simulink library "Actuator_Lib2"  (R2013a)
settings: Solver=ode45  StartTime=0.0  StopTime=10.0  RelTol=1e-3
values from neighbouring files (symbols this model uses):
  AC = FASER_config    [UAV_config.m]    (also in UAV_modelconfig.mat = )
  TrimCondition =     [UAV_trimcondition.mat]
undefined symbols (not defined in the file or in its folder): SampleTime
libraries: simulink x9, Actuator_Lib x6
settings Model: Creator=austinmurch  LastModifiedBy=descobar

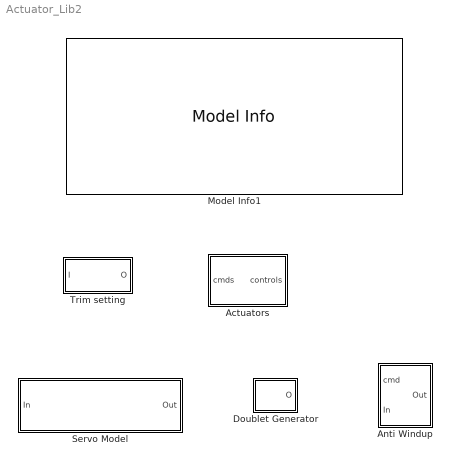
== system Actuator_Lib2 ==
  Actuators : Subsystem
  Anti Windup : Subsystem  mask(Integrator Anti-Windup){MAX_DEF=0, MIN_DEF=0, gain_sign=off}
      mask prompts: MAX_DEF "Maximum surface deflection limit"; MIN_DEF "Minimum surface deflection limit"; gain_sign "Positive gains in control law"
      mask help:
      | This block uses boolean logic to eliminate integrator windup.
      | It compares the sign of the error between reference and output,
      | and the sign and position of the surface being controlled.
      mask Help:
      | See the "READ ME" block under the mask for a more thorough explanation of
      | how this block works.
  Doublet Generator : Subsystem  mask(DoubletGenerator){timeon=[3 10 17], pulsewidth=[2 2 2], amplitude=[0 0 0]}
      mask prompts: timeon "Time Start"; pulsewidth "Pulse Duration"
      mask help:
      | Doublet Generator.
      | Ouputs doublet of specificed amplitude and duration.
      |
      | If start/duration/amplitude parameters are vectors, then output is multichannel.
      mask Display: plot([.1 .3 .3001 .4 .4001 .5  .5001 .7],[0 0 1 1 -1 -1 0 0])
  Model Info1 : simulink/Model-Wide Utilities/Model Info  InitialBlockCM=None  BlockCM=None  Frame=on  DisplayStringWithTags=|  HorizontalTextAlignment=Left  LeftAlignmentValue=0.02  SourceBlockDiagram=Actuator_Lib  TagMaxNumber=20
      | MODEL INFORMATION
      | Actuator Model Library
      | 
      | University of Minnesota
      | Aerospace Engineering and Mechanics
      | Copyright 2011 Regents of the University of Minnesota. All rights reserved.
      | 
      | == SVN Info ==
      | %<ModelVersion>
      | Last modified by %<LastModifiedBy> on %<LastModificationDate>
  Servo Model : Subsystem  mask(Rate and Position Limited Servo){freq=10, RL=999.0, POS_hi=20.0, POS_lo=-30.0}
      mask prompts: freq "Bandwidth, Hz"; RL "Rate Limit:"; POS_hi "Position Limit High:"; POS_lo "Position Limit Low:"
      mask help: First order transfer function: w/(s+w), with rate and position limits.
      mask Help:
      | This block models a first order servo with the initial condition
      | on the integrator set to the steady state value for constant input.
      | The servo is rate and position limited and those values are set
      | in the block parameters.
      mask Display:
      | text(.48,.55,sprintf('%3.1f Hz\nBW',freq),'horizontalAlignment','center');
      | 
      | text(0.18,0.45,sprintf('|d/dt|\n<%0.1f',RL),'horizontalAlignment','center');
      | 
      | text(0.88,0.85,num2str(POS_hi),'horizontalAlignment', 'center');
      | text(0.88,0.2,num2str(POS_lo),'horizontalAlignment', 'center');
      | text(0.73,0.5,'P\nL');
      | 
      | 
      | plot([0.83 0.87 0.93 0.97],[0.4 0.4 0.6 0.6]);
      | plot([0.81 0.99],[0.5 0.5]);
      | plot([0.9 0.9],[0.3 0.7]);
      | plot([0.81 0.99 0.99 0.81 0.81],[0.3 0.3 0.7 0.7 0.3]);
  "Trim setting " : Subsystem

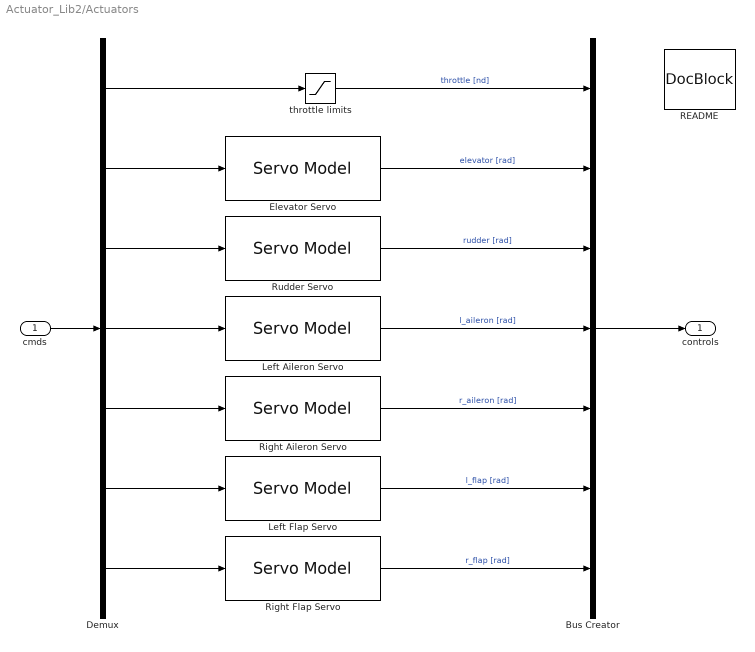
== system Actuator_Lib2/Actuators ==
  cmds : Inport
  Bus Creator : BusCreator  Inputs=7
  Demux : Demux  Outputs=7
  Elevator Servo : Actuator_Lib/Servo Model  freq=AC.Actuator.elevator.BW  RL=AC.Actuator.elevator.RateLim  POS_hi=AC.Actuator.elevator.PosLim  POS_lo=AC.Actuator.elevator.NegLim
  Left Aileron Servo : Actuator_Lib/Servo Model  freq=AC.Actuator.l_aileron.BW  RL=AC.Actuator.l_aileron.RateLim  POS_hi=AC.Actuator.l_aileron.PosLim  POS_lo=AC.Actuator.l_aileron.NegLim
  Left Flap Servo : Actuator_Lib/Servo Model  freq=AC.Actuator.l_flap.BW  RL=AC.Actuator.l_flap.RateLim  POS_hi=AC.Actuator.l_flap.PosLim  POS_lo=AC.Actuator.l_flap.NegLim
  README : simulink/Model-Wide Utilities/DocBlock  DocumentType=Text
      content=|
      | Actuators
      |
      | This block implements first order, rate and position limited actuator
      | models for the aileron, elevator, rudder and flap channels. The throttle
      | does not have a servo, but is position limited.
      |
      | Parameters for these models are contained in the aircraft configuration
      | data structure variable, "AC". Specfically,
      |
      | >> AC.Actuator
      |
      | ans =
      |
      |      elevator: [1x1 struct]
      |     l_aileron: [1x1 struct]
      |     r_aileron: [1x1 struct]
      |        rudder: [1x1 struct]
      |        l_flap: [1x1 struct]
      |        r_flap: [1x1 struct]
      |      throttle: [1x1 struct]
      |
      | Control Inputs Sign Convention
      | Elevator: +TED
      | Rudder: +TEL
      | Ailerons: +TED, da = (da_R-da_L)/2
      | Flaps: +TED
      | Throttle: always positive
  Right Aileron Servo : Actuator_Lib/Servo Model  freq=AC.Actuator.r_aileron.BW  RL=AC.Actuator.r_aileron.RateLim  POS_hi=AC.Actuator.r_aileron.PosLim  POS_lo=AC.Actuator.r_aileron.NegLim
  Right Flap Servo : Actuator_Lib/Servo Model  freq=AC.Actuator.l_flap.BW  RL=AC.Actuator.l_flap.RateLim  POS_hi=AC.Actuator.l_flap.PosLim  POS_lo=AC.Actuator.l_flap.NegLim
  Rudder Servo : Actuator_Lib/Servo Model  freq=AC.Actuator.rudder.BW  RL=AC.Actuator.rudder.RateLim  POS_hi=AC.Actuator.rudder.PosLim  POS_lo=AC.Actuator.rudder.NegLim
  throttle limits : Saturate  UpperLimit=AC.Actuator.throttle.PosLim  LowerLimit=AC.Actuator.throttle.NegLim
  controls : Outport
  wires:
  Demux/5 -> Right Aileron Servo/1
  Demux/7 -> Right Flap Servo/1
  Right Flap Servo/1 -> Bus Creator/7  "r_flap [rad]"
  Right Aileron Servo/1 -> Bus Creator/5  "r_aileron [rad]"
  Left Flap Servo/1 -> Bus Creator/6  "l_flap [rad]"
  Demux/6 -> Left Flap Servo/1
  Left Aileron Servo/1 -> Bus Creator/4  "l_aileron [rad]"
  Demux/4 -> Left Aileron Servo/1
  Rudder Servo/1 -> Bus Creator/3  "rudder [rad]"
  Demux/3 -> Rudder Servo/1
  Elevator Servo/1 -> Bus Creator/2  "elevator [rad]"
  Demux/2 -> Elevator Servo/1
  throttle limits/1 -> Bus Creator/1  "throttle [nd]"
  Demux/1 -> throttle limits/1
  cmds/1 -> Demux/1
  Bus Creator/1 -> controls/1

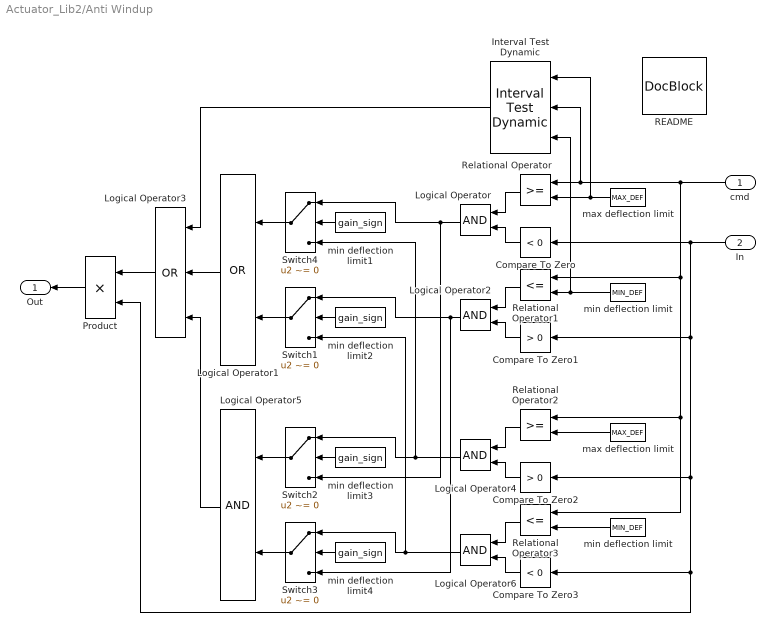
== system Actuator_Lib2/Anti Windup ==
  cmd : Inport
  In : Inport  Port=2
  Compare To Zero : simulink/Logic and Bit Operations/Compare To Zero  SystemSampleTime=-1  relop=<  LogicOutDataTypeMode=uint8
  Compare To Zero1 : simulink/Logic and Bit Operations/Compare To Zero  SystemSampleTime=-1  relop=>  LogicOutDataTypeMode=uint8
  Compare To Zero2 : simulink/Logic and Bit Operations/Compare To Zero  SystemSampleTime=-1  relop=>  LogicOutDataTypeMode=uint8
  Compare To Zero3 : simulink/Logic and Bit Operations/Compare To Zero  SystemSampleTime=-1  relop=<  LogicOutDataTypeMode=uint8
  Interval Test Dynamic : simulink/Logic and Bit Operations/Interval Test Dynamic  SystemSampleTime=-1  IntervalClosedRight=on  IntervalClosedLeft=on  LogicOutDataTypeMode=boolean
  Logical Operator{,2,4..6} (5 alike) : Logic  AllPortsSameDT=off  OutDataTypeStr=boolean  SampleTime=SampleTime
  Logical Operator1 : Logic  Operator=OR  AllPortsSameDT=off  OutDataTypeStr=boolean  SampleTime=SampleTime
  Logical Operator3 : Logic  Operator=OR  Inputs=3  AllPortsSameDT=off  OutDataTypeStr=boolean  SampleTime=SampleTime
  Product : Product  RndMeth=Zero
  README : simulink/Model-Wide Utilities/DocBlock  SystemSampleTime=-1  DocumentType=Text
      content=|
      | This block uses anti-windup logic to either stop or continue integrating.
      |
      | The first input signal, 'cmd', must come from the control surface command
      | that is the output of the controller. For instance, if the outputs of a PI
      | control phi tracker (with anti-windup) and a P control roll damper are
      | summed and sent to the aileron command, then the summed value must be fed
      | back into the 'cmd' input of this anti-windup block, as opposed to just the
      | output of the phi tracker.
      |
      | The second input signal, 'In', must come from the error that is being fed
      | into the control law.
      |
      | The output signal, 'Out' must feed into the error integrator block.
      |
      | For the anti-windup to work as intended, a saturation block must be placed
      | on the ouput of the control command being fed to the associated actuator.
      | If the controller is in delta coordinates, the limits in the saturation
      | block must be the actuator limits minus the trimmed control surface value.
      | For instance, for and aileron command, the limits would be:
      | Upper Limit: AC.Actuator.r_aileron.PosLim-TrimCondition.Inputs.r_aileron
      | Lower Limit: AC.Actuator.r_aileron.NegLim-TrimCondition.Inputs.r_aileron
      |
      | Depending on which surface is being controlled, the windup logic may
      | change. The default logic for this block is the following:
      |
      | For input u, saturation limits Umax and Umin, and error e,
      | If u is in bounds, do nothing
      | If u >= Umax AND e < 0, stop integrating
      | If u >= Umax AND e > 0, continue integrating
      | If u <= Umin AND e < 0, continue integrating
      | If u <= Umin AND e > 0, stop integrating
      |
      | This is the logic for a plant transfer function with a negative gain. In
      | other words, a positive input gives a negative response, which is usually
      | the case with flight dynamics. If the plant transfer function does not have
      | a negative gain, the logic will need to be reversed. In this case, the
      | inequalities on the error logic must be switched, so
      | If u is in bounds, do nothing
      | If u >= Umax AND e > 0, stop integrating
      | If u >= Umax AND e < 0, continue integrating
      | If u <= Umin AND e > 0, continue integrating
      | If u <= Umin AND e < 0, stop integrating
  Relational Operator : RelationalOperator  OutDataTypeStr=boolean
  Relational Operator1 : RelationalOperator  Operator=<=  OutDataTypeStr=boolean
  Relational Operator2 : RelationalOperator  OutDataTypeStr=boolean
  Relational Operator3 : RelationalOperator  Operator=<=  OutDataTypeStr=boolean
  Switch{1..4} (4 alike) : Switch  Criteria=u2 ~= 0  SampleTime=SampleTime
  max deflection limit : Constant  Value=MAX_DEF  SampleTime=SampleTime
  "max deflection limit " : Constant  Value=MAX_DEF  SampleTime=SampleTime
  min deflection limit : Constant  Value=MIN_DEF  SampleTime=SampleTime
  "min deflection limit " : Constant  Value=MIN_DEF  SampleTime=SampleTime
  min deflection limit{1..4} (4 alike) : Constant  Value=gain_sign  SampleTime=SampleTime
  Out : Outport
  wires:
  Logical Operator5/1 -> Logical Operator3/3
  "max deflection limit "/1 -> Relational Operator2/2
  "min deflection limit "/1 -> Relational Operator3/2
  Relational Operator3/1 -> Logical Operator6/1
  Compare To Zero3/1 -> Logical Operator6/2
  Relational Operator2/1 -> Logical Operator4/1
  Compare To Zero2/1 -> Logical Operator4/2
  Interval Test Dynamic/1 -> Logical Operator3/1
  Logical Operator1/1 -> Logical Operator3/2
  Logical Operator3/1 -> Product/1
  Product/1 -> Out/1
  min deflection limit/1 -> Interval Test Dynamic/3, Relational Operator1/2
  Relational Operator1/1 -> Logical Operator2/1
  Compare To Zero1/1 -> Logical Operator2/2
  In/1 -> Product/2, Compare To Zero3/1, Compare To Zero2/1, Compare To Zero1/1, Compare To Zero/1
  Relational Operator/1 -> Logical Operator/1
  Compare To Zero/1 -> Logical Operator/2
  cmd/1 -> Relational Operator3/1, Relational Operator2/1, Relational Operator1/1, Interval Test Dynamic/2, Relational Operator/1
  max deflection limit/1 -> Interval Test Dynamic/1, Relational Operator/2
  min deflection limit2/1 -> Switch1/2
  min deflection limit3/1 -> Switch2/2
  min deflection limit4/1 -> Switch3/2
  Switch2/1 -> Logical Operator5/1
  Switch3/1 -> Logical Operator5/2
  Switch1/1 -> Logical Operator1/2
  Switch4/1 -> Logical Operator1/1
  min deflection limit1/1 -> Switch4/2
  Logical Operator/1 -> Switch4/1, Switch2/3
  Logical Operator2/1 -> Switch1/1, Switch3/3
  Logical Operator4/1 -> Switch2/1, Switch4/3
  Logical Operator6/1 -> Switch3/1, Switch1/3

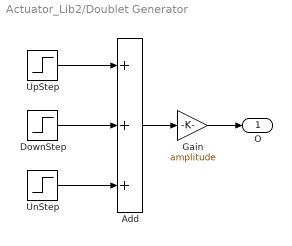
== system Actuator_Lib2/Doublet Generator ==
  Add : Sum  Inputs=+++
  DownStep : Step  Time=timeon+pulsewidth  After=-2  SampleTime=0
  Gain : Gain  Gain=amplitude
  UnStep : Step  Time=timeon+2*pulsewidth  SampleTime=0
  UpStep : Step  Time=timeon  SampleTime=0
  O : Outport
  wires:
  Gain/1 -> O/1
  Add/1 -> Gain/1
  UnStep/1 -> Add/3
  DownStep/1 -> Add/2
  UpStep/1 -> Add/1

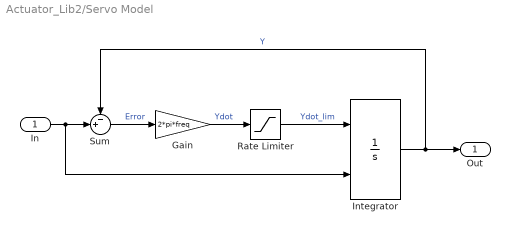
== system Actuator_Lib2/Servo Model ==
  In : Inport
  Gain : Gain  Gain=2*pi*freq  SaturateOnIntegerOverflow=on  OutDataTypeStr=Inherit: Same as input  ParamDataTypeStr=Inherit: Same as input
  Integrator : Integrator  InitialConditionSource=external  LimitOutput=on  UpperSaturationLimit=POS_hi  LowerSaturationLimit=POS_lo  IgnoreLimit=on
  Rate Limiter : Saturate  UpperLimit=RL  LowerLimit=-RL
  Sum : Sum  Inputs=-+|  SaturateOnIntegerOverflow=on  InputSameDT=on  OutDataTypeStr=Inherit: Same as first input
  Out : Outport  PortDimensions=1
  wires:
  Gain/1 -> Rate Limiter/1  "Ydot"
  Sum/1 -> Gain/1  "Error"
  Integrator/1 -> Sum/1, Out/1  "Y"
  Rate Limiter/1 -> Integrator/1  "Ydot_lim"
  In/1 -> Integrator/2, Sum/2

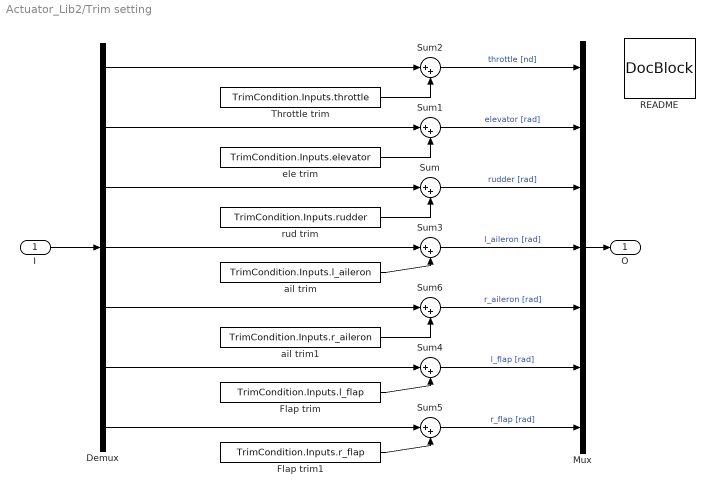
== system Actuator_Lib2/Trim setting  ==
  I : Inport
  Demux : Demux  Outputs=7
  Flap trim : Constant  Value=TrimCondition.Inputs.l_flap
  Flap trim1 : Constant  Value=TrimCondition.Inputs.r_flap
  Mux : Mux  Inputs=7
  README : simulink/Model-Wide Utilities/DocBlock  DocumentType=Text
      content=|
      | Trim Setting
      |
      | This block simply adds the trimmed control inputs to the control input. The
      | trimmed commands are contained in the TrimCondition data structure, in:
      |
      | >> TrimCondition.Inputs
      |
      | ans =
      |
      |            elevator: 0.0910
      |             aileron: 4.8789e-021
      |              rudder: -1.4404e-021
      |                flap: 0
      |            throttle: 0.5593
      |
      | Note even though there are physically two aileron servos and two flap
      | servos, the commands are treated as one here.
      |
      | The input command ordering must be:
      | aileron
      | elevator
      | rudder
      | throttle
      | flap
  Sum{,1..6} (7 alike) : Sum  Inputs=|++
  Throttle trim : Constant  Value=TrimCondition.Inputs.throttle
  ail trim : Constant  Value=TrimCondition.Inputs.l_aileron
  ail trim1 : Constant  Value=TrimCondition.Inputs.r_aileron
  ele trim : Constant  Value=TrimCondition.Inputs.elevator
  rud trim : Constant  Value=TrimCondition.Inputs.rudder
  O : Outport
  wires:
  Sum5/1 -> Mux/7  "r_flap [rad]"
  Sum4/1 -> Mux/6  "l_flap [rad]"
  Demux/5 -> Sum6/1
  Sum6/1 -> Mux/5  "r_aileron [rad]"
  ail trim1/1 -> Sum6/2
  Demux/6 -> Sum4/1
  Demux/7 -> Sum5/1
  Flap trim1/1 -> Sum5/2
  Demux/4 -> Sum3/1
  Sum3/1 -> Mux/4  "l_aileron [rad]"
  Sum/1 -> Mux/3  "rudder [rad]"
  Sum1/1 -> Mux/2  "elevator [rad]"
  Demux/1 -> Sum2/1
  ail trim/1 -> Sum3/2
  Sum2/1 -> Mux/1  "throttle [nd]"
  Throttle trim/1 -> Sum2/2
  rud trim/1 -> Sum/2
  Demux/3 -> Sum/1
  ele trim/1 -> Sum1/2
  I/1 -> Demux/1
  Demux/2 -> Sum1/1
  Flap trim/1 -> Sum4/2
  Mux/1 -> O/1
